simulink model "Lecture_1_Exercises"  (R2023b)
settings: Solver=VariableStepAuto  StartTime=0.0  StopTime=10.0  RelTol=1e-3
settings Model: Creator=Therkelsen  LastModifiedBy=Therkelsen

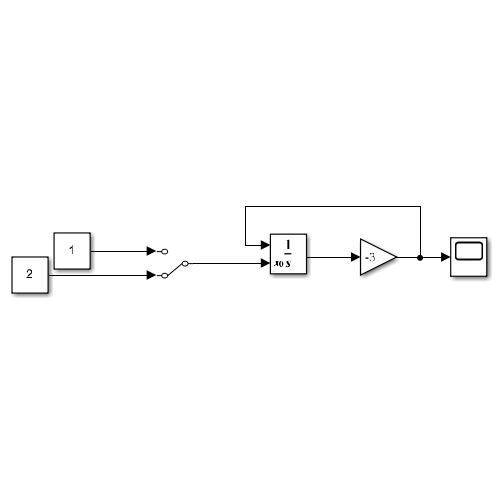
[thumbnail: Simulink's stored preview of the top-level diagram]
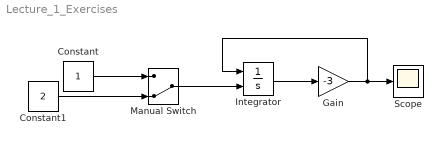
== system Lecture_1_Exercises ==
  Constant : Constant
  Constant1 : Constant  Value=2
  Gain : Gain  Gain=-3
  Integrator : Integrator  InitialConditionSource=external  InitialCondition=1
  Manual Switch : ManualSwitch  CurrentSetting=0
  Scope : Scope
  wires:
  Integrator/1 -> Gain/1
  Gain/1 -> Scope/1, Integrator/1
  Manual Switch/1 -> Integrator/2
  Constant/1 -> Manual Switch/1
  Constant1/1 -> Manual Switch/2
